simulink model "my_PLL_IntegerN_noiseless"  (R2024b)
settings: Solver=VariableStepAuto  StartTime=0.0  StopTime=10e-6  RelTol=1e-3
model workspace (MAT data in the model file):
  PhaseNoise_42 = [-191.261666509 -181.016259323 -185.62739633]
  PnFrequencyOffset_42 = [50000000 25000000 75000000]
  TargetFrequency_30 = 2100000000
  TargetPhaseNoise_30 = [-85 -125 -150 -180]
  phaseNoiseResultTable = [25000000  -181.016259323  -55; 50000000  -191.261666509  -45; 75000000  -185.62739633  -65]
  resolutionBandwidth = 30000
  uniqueStringPll_30 = '95_7167'
  uniqueString_41 = '91_3376'
  uniqueString_42 = '9_754'
libraries: msbPllFoundation x5
settings Model: VariantFading=off  Creator=BrunoFraga  LastModifiedBy=brunoalexandrefraga

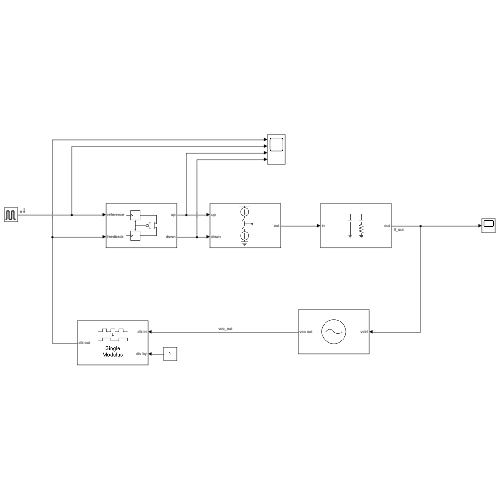
[thumbnail: Simulink's stored preview of the top-level diagram]
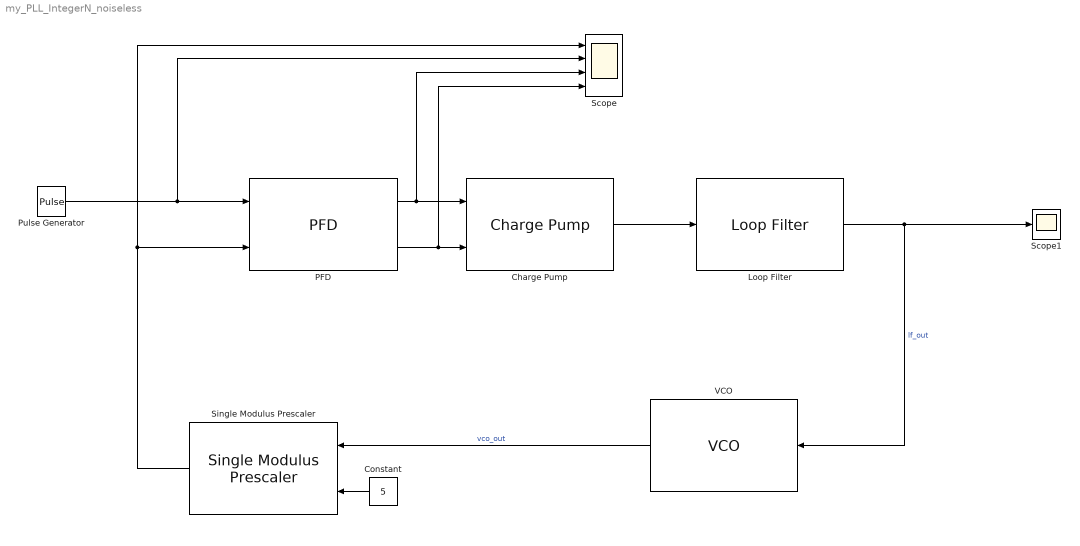
== system my_PLL_IntegerN_noiseless ==
  Charge Pump : msbPllFoundation/Charge Pump  OutputCurrent=1e-3  InputThreshold=0.5  ExtraBuffer=off  NBuffer=1000  EnableCurrentImpairments=off  CurrentImbalance=1e-4  LeakageCurrent=1e-5  EnableTimingImpairments=off  DefaultOrAdvanced=Default  MaxFreqInterest=10e9  RiseFallUp=50e-12  PropDelayUp=60e-12  RiseFallDown=20e-12  PropDelayDown=40e-12
  Constant : Constant  Value=5
  Loop Filter : msbPllFoundation/Loop Filter  FilterType=2nd order passive  C1=8.06e-11  C2=8.06e-10  C3=1.0452e-15  C4=1e-12  R2=2.79e+03  R3=51.0435e6  R4=12e3  ExtraBuffer=off  NBuffer=1000  EnableImpairments=off  Temperature=30
  PFD : msbPllFoundation/PFD  DeadbandCompensation=30e-12  ExtraBuffer=off  NBuffer=1000  EnableImpairments=off  DefaultOrAdvanced=Default  MaxFreqInterest=10e9  RiseFallTime=30e-12  PropDelay=50e-12
  Pulse Generator : DiscretePulseGenerator  PulseType=Time based  Period=1/10e6  PulseWidth=50
  Scope : Scope  NumInputPorts=4
  Scope1 : Scope
  Single Modulus Prescaler : msbPllFoundation/Single Modulus Prescaler  ExtraBuffer=off  NBuffer=1000
  VCO : msbPllFoundation/VCO  SpecifyUsing=Voltage sensitivity  Kvco=10e6  Fo=50e6  ControlVoltage=[-5 0 5]  OutputFrequency=[2e9 2.5e9 3e9]  Amplitude=1  ExtraBuffer=off  NBuffer=1000  AddPhaseNoise=off  Foffset=[10e3 100e3 1e6 3e6 10e6]  PhaseNoise=[-77 -108 -134 -145 -154]  MaxKvco=10000000
  wires:
  Pulse Generator/1 -> Scope/2, PFD/1
  VCO/1 -> Single Modulus Prescaler/1  "vco_out"
  Constant/1 -> Single Modulus Prescaler/2
  PFD/2 -> Scope/4, Charge Pump/2
  Charge Pump/1 -> Loop Filter/1
  PFD/1 -> Scope/3, Charge Pump/1
  Single Modulus Prescaler/1 -> Scope/1, PFD/2
  Loop Filter/1 -> VCO/1, Scope1/1  "lf_out"
